simulink model "d_009_2"  (Simulink 8.3)
settings: Solver=ode45  StartTime=0.0  StopTime=10.0  RelTol=1e-3
libraries: fm_lib x9
settings Model: Creator=fmilano  LastModifiedBy=F  ExtModeAutoUpdateStatusClock=off
settings OptimizationCC: BooleanDataType=off  InitFltsAndDblsToZero=on
settings DebuggingCC: SaveWithParameterizedLinksMsg=none  SignalResolutionControl=TryResolveAllWithWarning  SolverPrmCheckMsg=none  MultiTaskDSMMsg=warning  MultiTaskCondExecSysMsg=none  StateNameClashWarn=none  StrictBusMsg=None
settings HardwareCC: TargetUnknown=on
settings RTWCC: IncludeERTFirstTime=on
settings GRTTargetCC: TargetFcnLib=ansi_tfl_tmw.mat  CodeReplacementLibrary=ANSI_C  CompOptLevelCompliant=off  CPPClassGenCompliant=off

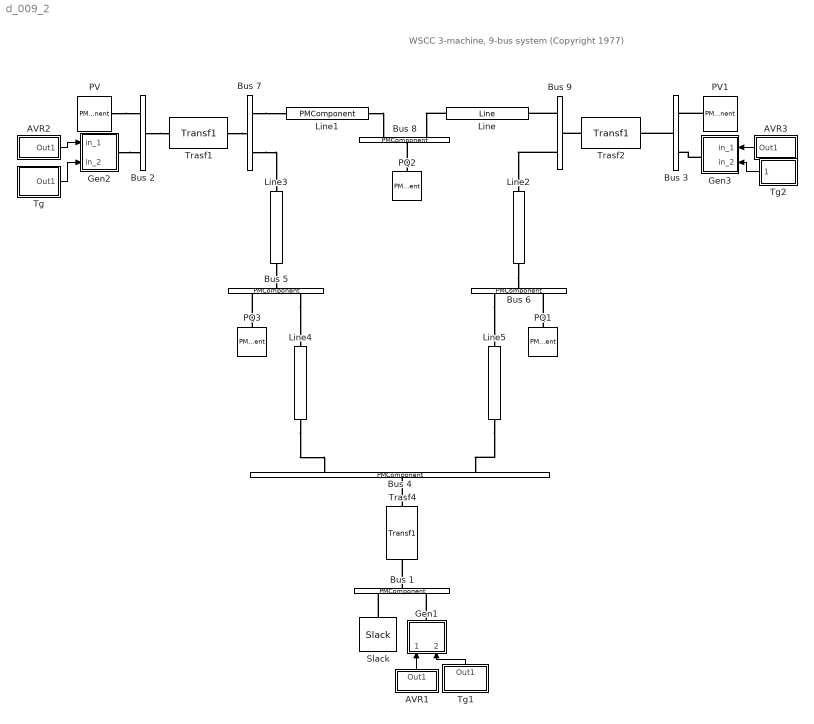
== system d_009_2 ==
  note: WSCC 3-machine, 9-bus system (Copyright 1977)
  AVR1 : Subsystem  Tag=PSATblock  Description=Controls  mask(Exc){p2q=2, p3q=5.00, p4q=-5.00, p5q=20, p6q=0.2, p7q=0.063, p8q=0.35, p9q=1, p10q=0.314, p11q=0.001, p12_13q=[0.0039  1.555], in=0}
      mask prompts: p2q "Automatic Voltage Regulator Type"; p3q "Maximum Regulator Voltage [p.u.]"; p4q "Minimum Regulator Voltage [p.u.]"; p5q "Amplifier Gain Ka [p.u./p.u.]"; p6q "Amplifier Time Constant Ta [s]"; p7q "Stabilizer Gain Kf [p.u./p.u.]"; p8q "Stabilizer Time Tf [s]"; p9q "Coefficient Kd [p.u./p.u.]"; p10q "Time Constant of the Field Circuit Td [s]"; p11q "Time Delay of the Measurement System Tr [s]"; p12_13q "Coefficient of the Ceiling Function (A B)"; in "Number of input signals"
      mask help: This block defines an Automatic Voltage Regulator.
      mask init:
      | fm_inout
      | [x,y] = fm_draw('R');
      mask Help:
      | This block defines an Automatic Voltage Regulator.
      | There are three kind of regulators:
      | 
      | Type 1:
      | 
      |      IEEE Model 1
      | 
      | Type 2:
      | 
      |      IEEE Model 2
      | 
      | Type 3:
      | 
      |      IEEE Model 3
      mask TypeOptions p2q: 1 | 2 | 3
      mask Callback p2q: fm_block
      mask TypeOptions in: 0 | 1 | 2 | 3
      mask Display:
      | plot([-1.8 4.1 4.1 -1.8 -1.8],[-1.5 -1.5 1.5 1.5 -1.5])
      | color('red')
      | plot([-1.3 -0.5],[-1 1],[-0.5 0.3],[1 -1],[-0.9 -0.1],[0.0 0.0])
      | plot(2.8+1.3*x,2*y,1.5+[-1.3 -0.5],[1 -1],1.5+[-0.5 0.3],[-1 1])
  AVR2 : Subsystem  Tag=PSATblock  Description=Controls  mask(Exc){p2q=2, p3q=5.00, p4q=-5.00, p5q=20, p6q=0.2, p7q=0.063, p8q=0.35, p9q=1, p10q=0.314, p11q=0.001, p12_13q=[0.0039  1.555], in=0}
      mask prompts: p2q "Automatic Voltage Regulator Type"; p3q "Maximum Regulator Voltage [p.u.]"; p4q "Minimum Regulator Voltage [p.u.]"; p5q "Amplifier Gain Ka [p.u./p.u.]"; p6q "Amplifier Time Constant Ta [s]"; p7q "Stabilizer Gain Kf [p.u./p.u.]"; p8q "Stabilizer Time Tf [s]"; p9q "Coefficient Kd [p.u./p.u.]"; p10q "Time Constant of the Field Circuit Td [s]"; p11q "Time Delay of the Measurement System Tr [s]"; p12_13q "Coefficient of the Ceiling Function (A B)"; in "Number of input signals"
      mask help: This block defines an Automatic Voltage Regulator.
      mask init:
      | fm_inout
      | [x,y] = fm_draw('R');
      mask Help:
      | This block defines an Automatic Voltage Regulator.
      | There are three kind of regulators:
      | 
      | Type 1:
      | 
      |      IEEE Model 1
      | 
      | Type 2:
      | 
      |      IEEE Model 2
      | 
      | Type 3:
      | 
      |      IEEE Model 3
      mask TypeOptions p2q: 1 | 2 | 3
      mask Callback p2q: fm_block
      mask TypeOptions in: 0 | 1 | 2 | 3
      mask Display:
      | plot([-1.8 4.1 4.1 -1.8 -1.8],[-1.5 -1.5 1.5 1.5 -1.5])
      | color('red')
      | plot([-1.3 -0.5],[-1 1],[-0.5 0.3],[1 -1],[-0.9 -0.1],[0.0 0.0])
      | plot(2.8+1.3*x,2*y,1.5+[-1.3 -0.5],[1 -1],1.5+[-0.5 0.3],[-1 1])
  AVR3 : Subsystem  Tag=PSATblock  Description=Controls  mask(Exc){p2q=2, p3q=5.00, p4q=-5.00, p5q=20, p6q=0.2, p7q=0.063, p8q=0.35, p9q=1, p10q=0.314, p11q=0.001, p12_13q=[0.0039  1.555], in=0}
      mask prompts: p2q "Automatic Voltage Regulator Type"; p3q "Maximum Regulator Voltage [p.u.]"; p4q "Minimum Regulator Voltage [p.u.]"; p5q "Amplifier Gain Ka [p.u./p.u.]"; p6q "Amplifier Time Constant Ta [s]"; p7q "Stabilizer Gain Kf [p.u./p.u.]"; p8q "Stabilizer Time Tf [s]"; p9q "Coefficient Kd [p.u./p.u.]"; p10q "Time Constant of the Field Circuit Td [s]"; p11q "Time Delay of the Measurement System Tr [s]"; p12_13q "Coefficient of the Ceiling Function (A B)"; in "Number of input signals"
      mask help: This block defines an Automatic Voltage Regulator.
      mask init:
      | fm_inout
      | [x,y] = fm_draw('R');
      mask Help:
      | This block defines an Automatic Voltage Regulator.
      | There are three kind of regulators:
      | 
      | Type 1:
      | 
      |      IEEE Model 1
      | 
      | Type 2:
      | 
      |      IEEE Model 2
      | 
      | Type 3:
      | 
      |      IEEE Model 3
      mask TypeOptions p2q: 1 | 2 | 3
      mask Callback p2q: fm_block
      mask TypeOptions in: 0 | 1 | 2 | 3
      mask Display:
      | plot([-1.8 4.1 4.1 -1.8 -1.8],[-1.5 -1.5 1.5 1.5 -1.5])
      | color('red')
      | plot([-1.3 -0.5],[-1 1],[-0.5 0.3],[1 -1],[-0.9 -0.1],[0.0 0.0])
      | plot(2.8+1.3*x,2*y,1.5+[-1.3 -0.5],[1 -1],1.5+[-0.5 0.3],[-1 1])
  Bus 1 : PMComponent  Tag=PSATblock  Description=Connection  PhysicalDomain=psatdomain  LeftPortType=p1  RightPortType=p1  LConnTagsString=__newl0|__newl1  RConnTagsString=__newr0  mask(Bus){in=2, out=1, p2q=16.5, p3_4q=[1.00   0.00], p5q=4, p6q=1}
      mask prompts: in "Number of inputs:"; out "Number of outputs:"; p2q "Voltage Rating [kV]"; p3_4q "Voltage initial guess [p.u.  rad]"; p5q "Area number"; p6q "Region number"
      mask help: Bus block.
      mask init:
      | fm_inout
      mask Callback p5q: fm_block
      mask Display: plot([0 1 1 0 0],[0 0 1 1 0])
  Bus 2 : PMComponent  Tag=PSATblock  Description=Connection  PhysicalDomain=psatdomain  LeftPortType=p1  RightPortType=p1  LConnTagsString=__newl0|__newl1  RConnTagsString=__newr0  mask(Bus){in=2, out=1, p2q=18, p3_4q=[1.00   0.00], p5q=5, p6q=1}
      mask prompts: in "Number of inputs:"; out "Number of outputs:"; p2q "Voltage Rating [kV]"; p3_4q "Voltage initial guess [p.u.  rad]"; p5q "Area number"; p6q "Region number"
      mask help: Bus block.
      mask init:
      | fm_inout
      mask Callback p5q: fm_block
      mask Display: plot([0 1 1 0 0],[0 0 1 1 0])
  Bus 3 : PMComponent  Tag=PSATblock  Description=Connection  PhysicalDomain=psatdomain  LeftPortType=p1  RightPortType=p1  LConnTagsString=__newl0|__newl1  RConnTagsString=__newr0  mask(Bus){in=2, out=1, p2q=13.8, p3_4q=[1.00   0.00], p5q=3, p6q=1}
      mask prompts: in "Number of inputs:"; out "Number of outputs:"; p2q "Voltage Rating [kV]"; p3_4q "Voltage initial guess [p.u.  rad]"; p5q "Area number"; p6q "Region number"
      mask help: Bus block.
      mask init:
      | fm_inout
      mask Callback p5q: fm_block
      mask Display: plot([0 1 1 0 0],[0 0 1 1 0])
  Bus 4 : PMComponent  Tag=PSATblock  Description=Connection  PhysicalDomain=psatdomain  LeftPortType=p1  RightPortType=p1  LConnTagsString=__newl0|__newl1  RConnTagsString=__newr0  mask(Bus){in=2, out=1, p2q=230, p3_4q=[1.00   0.00], p5q=2, p6q=1}
      mask prompts: in "Number of inputs:"; out "Number of outputs:"; p2q "Voltage Rating [kV]"; p3_4q "Voltage initial guess [p.u.  rad]"; p5q "Area number"; p6q "Region number"
      mask help: Bus block.
      mask init:
      | fm_inout
      mask Callback p5q: fm_block
      mask Display: plot([0 1 1 0 0],[0 0 1 1 0])
  Bus 5 : PMComponent  Tag=PSATblock  Description=Connection  PhysicalDomain=psatdomain  LeftPortType=p1  RightPortType=p1  LConnTagsString=__newl0  RConnTagsString=__newr0|__newr1  mask(Bus){in=1, out=2, p2q=230, p3_4q=[1.00   0.00], p5q=2, p6q=1}
      mask prompts: in "Number of inputs:"; out "Number of outputs:"; p2q "Voltage Rating [kV]"; p3_4q "Voltage initial guess [p.u.  rad]"; p5q "Area number"; p6q "Region number"
      mask help: Bus block.
      mask init:
      | fm_inout
      mask Callback p5q: fm_block
      mask Display: plot([0 1 1 0 0],[0 0 1 1 0])
  Bus 6 : PMComponent  Tag=PSATblock  Description=Connection  PhysicalDomain=psatdomain  LeftPortType=p1  RightPortType=p1  LConnTagsString=__newl0  RConnTagsString=__newr0|__newr1  mask(Bus){in=1, out=2, p2q=230, p3_4q=[1.00   0.00], p5q=2, p6q=1}
      mask prompts: in "Number of inputs:"; out "Number of outputs:"; p2q "Voltage Rating [kV]"; p3_4q "Voltage initial guess [p.u.  rad]"; p5q "Area number"; p6q "Region number"
      mask help: Bus block.
      mask init:
      | fm_inout
      mask Callback p5q: fm_block
      mask Display: plot([0 1 1 0 0],[0 0 1 1 0])
  Bus 7 : PMComponent  Tag=PSATblock  Description=Connection  PhysicalDomain=psatdomain  LeftPortType=p1  RightPortType=p1  LConnTagsString=__newl0  RConnTagsString=__newr0|__newr1  mask(Bus){in=1, out=2, p2q=230, p3_4q=[1.00   0.00], p5q=2, p6q=1}
      mask prompts: in "Number of inputs:"; out "Number of outputs:"; p2q "Voltage Rating [kV]"; p3_4q "Voltage initial guess [p.u.  rad]"; p5q "Area number"; p6q "Region number"
      mask help: Bus block.
      mask init:
      | fm_inout
      mask Callback p5q: fm_block
      mask Display: plot([0 1 1 0 0],[0 0 1 1 0])
  Bus 8 : PMComponent  Tag=PSATblock  Description=Connection  PhysicalDomain=psatdomain  LeftPortType=p1  RightPortType=p1  LConnTagsString=__newl0|__newl1  RConnTagsString=__newr0  mask(Bus){in=2, out=1, p2q=230, p3_4q=[1.00   0.00], p5q=2, p6q=1}
      mask prompts: in "Number of inputs:"; out "Number of outputs:"; p2q "Voltage Rating [kV]"; p3_4q "Voltage initial guess [p.u.  rad]"; p5q "Area number"; p6q "Region number"
      mask help: Bus block.
      mask init:
      | fm_inout
      mask Callback p5q: fm_block
      mask Display: plot([0 1 1 0 0],[0 0 1 1 0])
  Bus 9 : PMComponent  Tag=PSATblock  Description=Connection  PhysicalDomain=psatdomain  LeftPortType=p1  RightPortType=p1  LConnTagsString=__newl0  RConnTagsString=__newr0|__newr1  mask(Bus){in=1, out=2, p2q=230, p3_4q=[1.00   0.00], p5q=2, p6q=1}
      mask prompts: in "Number of inputs:"; out "Number of outputs:"; p2q "Voltage Rating [kV]"; p3_4q "Voltage initial guess [p.u.  rad]"; p5q "Area number"; p6q "Region number"
      mask help: Bus block.
      mask init:
      | fm_inout
      mask Callback p5q: fm_block
      mask Display: plot([0 1 1 0 0],[0 0 1 1 0])
  Gen1 : Subsystem  Tag=PSATblock  Description=Machines  mask(Syn){p2_3_4q=[100  16.5   60], p5q=4, p7_6q=[0.00  0.00], p8_9_10q=[0.1460  0.0608  0.0000], p11_12q=[8.96  0.00], p13_14_15q=[0.0969  0.0969  0.0000], p16_17q=[0.310  0.0000], p18_19q=[22  0.00], p20_21q=[0.00  0.00], p22_23q=[1.00  1.00], p24q=0.002, p25_26q=[0 0], in=2, p27q=1, p28q=on}
      mask prompts: p2_3_4q "Power, voltage and frequency ratings [MVA, kV, Hz]"; p5q "Machine Dynamic Order"; p7_6q "resistance ra and leakage reactance xl [p.u. p.u.]"; p8_9_10q "d-axis reactances Xd, X'd X"d [p.u.,p.u.,p.u.]"; p11_12q "d-axis open circuit time constants T'd0 and T"d0 [s, s]"; p13_14_15q "q-axis reactances Xq, X'q, X"q [p.u.  p.u.  p.u.]"; p16_17q "q-axis open circuit time constants T'q0 and T"q0 [s s]"; p18_19q "Inertia (M = 2H) and Damping [s, p.u.]"; p20_21q "Speed and active power additional signals Kw and Kp [p.u., p.u.]"; p22_23q "Percentage of active and reactive powers at bus [p.u. p.u.]"; p24q "d-axis additional circuit leakage time constant Taa [s]"; p25_26q "Saturation coefficients S(1.0) and S(1.2)"; in "Number of input signals"; p27q "COI number"; p28q "Connected"
      mask help: This block defines a fourth order synchronous machine.
      mask init:
      | fm_inout
      | [x,y] = fm_draw('circle');
      | [xg,yg] = fm_draw('G');
      | [xs,ys] = fm_draw('sinus');
      mask TypeOptions p5q: 8 | 6 | 5.3 | 5.2 | 5.1 | 4 | 3 | 2
      mask Callback p5q: fm_block
      mask TypeOptions in: 0 | 1 | 2
      mask Callback p28q: fm_block
      mask Display:
      | plot(x+1.4,y,0.12*xs+1,0.15*ys-0.6)
      | color('blue')
      | plot(1.4+0.45*xg,0.3+0.45*yg)
  Gen2 : Subsystem  Tag=PSATblock  Description=Machines  mask(Syn){p2_3_4q=[100  18   60], p5q=4, p7_6q=[0.00  0.00], p8_9_10q=[0.8958  0.1198  0.0000], p11_12q=[6.00  0.00], p13_14_15q=[0.8645  0.1969  0.0000], p16_17q=[0.5350  0.0000], p18_19q=[22  0.00], p20_21q=[0.00  0.00], p22_23q=[1.00  1.00], p24q=0.002, p25_26q=[0 0], in=2, p27q=1, p28q=on}
      mask prompts: p2_3_4q "Power, voltage and frequency ratings [MVA, kV, Hz]"; p5q "Machine Dynamic Order"; p7_6q "resistance ra and leakage reactance xl [p.u. p.u.]"; p8_9_10q "d-axis reactances Xd, X'd X"d [p.u.,p.u.,p.u.]"; p11_12q "d-axis open circuit time constants T'd0 and T"d0 [s, s]"; p13_14_15q "q-axis reactances Xq, X'q, X"q [p.u.  p.u.  p.u.]"; p16_17q "q-axis open circuit time constants T'q0 and T"q0 [s s]"; p18_19q "Inertia (M = 2H) and Damping [s, p.u.]"; p20_21q "Speed and active power additional signals Kw and Kp [p.u., p.u.]"; p22_23q "Percentage of active and reactive powers at bus [p.u. p.u.]"; p24q "d-axis additional circuit leakage time constant Taa [s]"; p25_26q "Saturation coefficients S(1.0) and S(1.2)"; in "Number of input signals"; p27q "COI number"; p28q "Connected"
      mask help: This block defines a fourth order synchronous machine.
      mask init:
      | fm_inout
      | [x,y] = fm_draw('circle');
      | [xg,yg] = fm_draw('G');
      | [xs,ys] = fm_draw('sinus');
      mask TypeOptions p5q: 8 | 6 | 5.3 | 5.2 | 5.1 | 4 | 3 | 2
      mask Callback p5q: fm_block
      mask TypeOptions in: 0 | 1 | 2
      mask Callback p28q: fm_block
      mask Display:
      | plot(x+1.4,y,0.12*xs+1,0.15*ys-0.6)
      | color('blue')
      | plot(1.4+0.45*xg,0.3+0.45*yg)
  Gen3 : Subsystem  Tag=PSATblock  Description=Machines  mask(Syn){p2_3_4q=[100  13.8   60], p5q=4, p7_6q=[0.00  0.00], p8_9_10q=[1.3125  0.1813  0.0000], p11_12q=[5.89  0.00], p13_14_15q=[1.2578  0.2500  0.0000], p16_17q=[0.600  0.0000], p18_19q=[4.4  0.00], p20_21q=[0.00  0.00], p22_23q=[1.00  1.00], p24q=0.002, p25_26q=[0 0], in=2, p27q=1, p28q=on}
      mask prompts: p2_3_4q "Power, voltage and frequency ratings [MVA, kV, Hz]"; p5q "Machine Dynamic Order"; p7_6q "resistance ra and leakage reactance xl [p.u. p.u.]"; p8_9_10q "d-axis reactances Xd, X'd X"d [p.u.,p.u.,p.u.]"; p11_12q "d-axis open circuit time constants T'd0 and T"d0 [s, s]"; p13_14_15q "q-axis reactances Xq, X'q, X"q [p.u.  p.u.  p.u.]"; p16_17q "q-axis open circuit time constants T'q0 and T"q0 [s s]"; p18_19q "Inertia (M = 2H) and Damping [s, p.u.]"; p20_21q "Speed and active power additional signals Kw and Kp [p.u., p.u.]"; p22_23q "Percentage of active and reactive powers at bus [p.u. p.u.]"; p24q "d-axis additional circuit leakage time constant Taa [s]"; p25_26q "Saturation coefficients S(1.0) and S(1.2)"; in "Number of input signals"; p27q "COI number"; p28q "Connected"
      mask help: This block defines a fourth order synchronous machine.
      mask init:
      | fm_inout
      | [x,y] = fm_draw('circle');
      | [xg,yg] = fm_draw('G');
      | [xs,ys] = fm_draw('sinus');
      mask TypeOptions p5q: 8 | 6 | 5.3 | 5.2 | 5.1 | 4 | 3 | 2
      mask Callback p5q: fm_block
      mask TypeOptions in: 0 | 1 | 2
      mask Callback p28q: fm_block
      mask Display:
      | plot(x+1.4,y,0.12*xs+1,0.15*ys-0.6)
      | color('blue')
      | plot(1.4+0.45*xg,0.3+0.45*yg)
  Line : fm_lib/Power Flow/Line  Tag=PSATblock  Description=Power Flow  LConnTagsString=__newl0  RConnTagsString=__newr0  p3_4_5q="[100  230  60]"  p6q=0  p8q=0.0119  p9q=0.1008  p10q=0.1045*2  p13_14_15q="[0.0  0.0  0.0]"  p16q=on
  Line1 : PMComponent  Tag=PSATblock  Description=Power Flow  PhysicalDomain=psatdomain  LeftPortType=p1  RightPortType=p1  LConnTagsString=__newl0  RConnTagsString=__newr0  mask(Line){p3_4_5q=[100  230  60], p6q=0, p8q=0.0085, p9q=0.072, p10q=0.0745*2, p13_14_15q=[0.0  0.0  0.0], p16q=on}
      mask prompts: p3_4_5q "Power, Voltage and Frequency Ratings [MVA, kV, Hz]"; p6q "Length of line [km] (0 for p.u. parameters)"; p8q "Resistance [p.u. (Ohms/km)]"; p9q "Reactance [p.u. (H/km)]"; p10q "Susceptance [p.u. (F/km)]"; p13_14_15q "Imax, Pmax and Smax [p.u., p.u., p.u.]"; p16q "Connected"
      mask help: This block defines a pi model for a tree phase line.
      mask init:
      | [xp,yp] = fm_draw('pi');
      mask Callback p16q: fm_block
      mask Display:
      | plot([-1  1  1 -1 -1],[-0.2 -0.2 0.2 0.2 -0.2])
      | color('blue')
      | plot(0.35*xp,0.2*yp)
  Line2 : fm_lib/Power Flow/Line  Tag=PSATblock  Description=Power Flow  LConnTagsString=__newl0  RConnTagsString=__newr0  p3_4_5q="[100  230  60]"  p6q=0  p8q=0.039  p9q=0.170  p10q=0.179*2  p13_14_15q="[0.0  0.0  0.0]"  p16q=on
  Line3 : fm_lib/Power Flow/Line  Tag=PSATblock  Description=Power Flow  LConnTagsString=__newl0  RConnTagsString=__newr0  p3_4_5q="[100  230  60]"  p6q=0  p8q=0.032  p9q=0.161  p10q=0.153*2  p13_14_15q="[0.0  0.0  0.0]"  p16q=on
  Line4 : fm_lib/Power Flow/Line  Tag=PSATblock  Description=Power Flow  LConnTagsString=__newl0  RConnTagsString=__newr0  p3_4_5q="[100  230  60]"  p6q=0  p8q=0.01  p9q=0.085  p10q=0.088*2  p13_14_15q="[0.0  0.0  0.0]"  p16q=on
  Line5 : fm_lib/Power Flow/Line  Tag=PSATblock  Description=Power Flow  LConnTagsString=__newl0  RConnTagsString=__newr0  p3_4_5q="[100  230  60]"  p6q=0  p8q=0.017  p9q=0.092  p10q=0.079*2  p13_14_15q="[0.0  0.0  0.0]"  p16q=on
  PQ1 : PMComponent  Tag=PSATblock  Description=Power Flow  PhysicalDomain=psatdomain  LeftPortType=p1  RightPortType=p1  LConnTagsString=__newl0  mask(PQ){p2_3q=[100  230], p4_5q=[0.9  0.3], p6_7q=[1.2  0.8], p8q=off, p9q=on}
      mask prompts: p2_3q "Power and Voltage Ratings [MVA, kV]"; p4_5q "Active and Reactive Powers [p.u.  p.u.]"; p6_7q "Maximum and Minimum Allowable Voltage [p.u.   p.u.]"; p8q "Allow conversion to impendance for min & max voltage"; p9q "Connected"
      mask help:
      | This block defines a constant power load:
      |
      | P = Pcost.
      | Q = Qcost.
      mask Callback p8q: fm_block
      mask Callback p9q: fm_block
      mask Display: plot([1 -0.5 -0.5 1],[0 0.866 -0.866 0])
  PQ2 : PMComponent  Tag=PSATblock  Description=Power Flow  PhysicalDomain=psatdomain  LeftPortType=p1  RightPortType=p1  LConnTagsString=__newl0  mask(PQ){p2_3q=[100  230], p4_5q=[1  0.35], p6_7q=[1.2  0.8], p8q=off, p9q=on}
      mask prompts: p2_3q "Power and Voltage Ratings [MVA, kV]"; p4_5q "Active and Reactive Powers [p.u.  p.u.]"; p6_7q "Maximum and Minimum Allowable Voltage [p.u.   p.u.]"; p8q "Allow conversion to impendance for min & max voltage"; p9q "Connected"
      mask help:
      | This block defines a constant power load:
      |
      | P = Pcost.
      | Q = Qcost.
      mask Callback p8q: fm_block
      mask Callback p9q: fm_block
      mask Display: plot([1 -0.5 -0.5 1],[0 0.866 -0.866 0])
  PQ3 : PMComponent  Tag=PSATblock  Description=Power Flow  PhysicalDomain=psatdomain  LeftPortType=p1  RightPortType=p1  LConnTagsString=__newl0  mask(PQ){p2_3q=[100  230], p4_5q=[1.25  0.5], p6_7q=[1.2  0.8], p8q=off, p9q=on}
      mask prompts: p2_3q "Power and Voltage Ratings [MVA, kV]"; p4_5q "Active and Reactive Powers [p.u.  p.u.]"; p6_7q "Maximum and Minimum Allowable Voltage [p.u.   p.u.]"; p8q "Allow conversion to impendance for min & max voltage"; p9q "Connected"
      mask help:
      | This block defines a constant power load:
      |
      | P = Pcost.
      | Q = Qcost.
      mask Callback p8q: fm_block
      mask Callback p9q: fm_block
      mask Display: plot([1 -0.5 -0.5 1],[0 0.866 -0.866 0])
  PV : PMComponent  Tag=PSATblock  Description=Power Flow  PhysicalDomain=psatdomain  LeftPortType=p1  RightPortType=p1  RConnTagsString=__newr0  mask(PV){p2_3q=[100  18], p4q=1.316, p5q=1.025, p6_7q=[99 -99], p8_9q=[1.1  0.9], p10q=1, p11q=on}
      mask prompts: p2_3q "Power and Voltage Ratings [MVA, kV]"; p4q "Active Power [p.u.]"; p5q "Voltage Magnitude [p.u.]"; p6_7q "Qmax and Qmin [p.u.  p.u.]"; p8_9q "Vmax and Vmin [p.u.  p.u.]"; p10q "Loss Participation Factor"; p11q "Connected"
      mask help:
      | This block defines a PV bus for load flow studies:
      |
      | P = Pcost.
      | V = Vdes.
      mask init:
      | [x,y] = fm_draw('circle');
      | [xp,yp] = fm_draw('P');
      mask Callback p11q: fm_block
      mask Display:
      | plot(x,y)
      | color('blue')
      | plot(0.3*xp-0.35,0.6*yp,[0.1 0.3 0.5],[0.3 -0.3 0.3])
  PV1 : PMComponent  Tag=PSATblock  Description=Power Flow  PhysicalDomain=psatdomain  LeftPortType=p1  RightPortType=p1  RConnTagsString=__newr0  mask(PV){p2_3q=[100  13.8], p4q=1.162, p5q=1.025, p6_7q=[99  -99], p8_9q=[1.1  0.9], p10q=1, p11q=on}
      mask prompts: p2_3q "Power and Voltage Ratings [MVA, kV]"; p4q "Active Power [p.u.]"; p5q "Voltage Magnitude [p.u.]"; p6_7q "Qmax and Qmin [p.u.  p.u.]"; p8_9q "Vmax and Vmin [p.u.  p.u.]"; p10q "Loss Participation Factor"; p11q "Connected"
      mask help:
      | This block defines a PV bus for load flow studies:
      |
      | P = Pcost.
      | V = Vdes.
      mask init:
      | [x,y] = fm_draw('circle');
      | [xp,yp] = fm_draw('P');
      mask Callback p11q: fm_block
      mask Display:
      | plot(x,y)
      | color('blue')
      | plot(0.3*xp-0.35,0.6*yp,[0.1 0.3 0.5],[0.3 -0.3 0.3])
  Slack : fm_lib/Power Flow/Slack  Tag=PSATblock  Description=Power Flow  RConnTagsString=__newr0  p2_3q="[100  16.5]"  p4q=1.04  p5q=0.00  p6_7q=[99 -99]  p8_9q="[1.1  0.9]"  p10q=0.80  p11q=1  p12q=on  p13q=on
  Tg : Subsystem  Tag=PSATblock  Description=Controls  mask(Tg){p2q=2, p3q=1.00, p4q=0.2, p5q=10, p6q=0.0, p7q=0.10, p8q=-0.10, p9q=0.04, p10q=5.0, p11q=0.04, p12q=0.3, p13q=1.0, p14q=0.5, p15q=1.0, p16q=1.5, p17q=1.0, p18q=1.163, p19q=0.105, p20q=on}
      mask prompts: p2q "Turbine governor type"; p3q "Reference speed [p.u.]"; p4q "Droop R [p.u.]"; p5q "Maximum torque [p.u.]"; p6q "Minimum torque [p.u.]"; p7q "Pole Time Constant T2 [s]"; p8q "Zero Time Constant T1 [s]"; p9q "Pilot valve time constant Tp [s]"; p10q "Dashpot time constant Tr [s]"; p11q "Permanent speed droop sigma [p.u./p.u.]"; p12q "Transient speed droop delta [p.u./p.u.]"; p13q "Water starting time Tw [s]"; p14q "Derivative of flow rate with respect to tubine head a11"; p15q "Derivative of flow rate with respect to gate position a13"; p16q "Derivative of torque with respect to tubine head a21"; p17q "Derivative of torque with respect to gate position a23"; p18q "Proportional droop Kp [p.u./p.u.]"; p19q "Integral droop Ki [p.u./p.u.]"; p20q "Connected"
      mask help: This block defines a Turbine Governor.
      mask init:
      | [x,y] = fm_draw('G');
      mask TypeOptions p2q: 1 | 2 | 3 | 4 | 5 | 6
      mask Callback p2q: fm_block
      mask Callback p20q: fm_block
      mask Display:
      | plot([-1.8 2.8 2.8 -1.8 -1.8],[-1.5 -1.5 1.5 1.5 -1.5])
      | color('red')
      | plot([-0.5 -0.5],[-1 1],[-1.3 0.3],[1 1])
      | plot(1.4+x,y)
  Tg1 : Subsystem  Tag=PSATblock  Description=Controls  mask(Tg){p2q=2, p3q=1.00, p4q=0.2, p5q=10, p6q=0.0, p7q=0.10, p8q=-0.10, p9q=0.04, p10q=5.0, p11q=0.04, p12q=0.3, p13q=1.0, p14q=0.5, p15q=1.0, p16q=1.5, p17q=1.0, p18q=1.163, p19q=0.105, p20q=on}
      mask prompts: p2q "Turbine governor type"; p3q "Reference speed [p.u.]"; p4q "Droop R [p.u.]"; p5q "Maximum torque [p.u.]"; p6q "Minimum torque [p.u.]"; p7q "Pole Time Constant T2 [s]"; p8q "Zero Time Constant T1 [s]"; p9q "Pilot valve time constant Tp [s]"; p10q "Dashpot time constant Tr [s]"; p11q "Permanent speed droop sigma [p.u./p.u.]"; p12q "Transient speed droop delta [p.u./p.u.]"; p13q "Water starting time Tw [s]"; p14q "Derivative of flow rate with respect to tubine head a11"; p15q "Derivative of flow rate with respect to gate position a13"; p16q "Derivative of torque with respect to tubine head a21"; p17q "Derivative of torque with respect to gate position a23"; p18q "Proportional droop Kp [p.u./p.u.]"; p19q "Integral droop Ki [p.u./p.u.]"; p20q "Connected"
      mask help: This block defines a Turbine Governor.
      mask init:
      | [x,y] = fm_draw('G');
      mask TypeOptions p2q: 1 | 2 | 3 | 4 | 5 | 6
      mask Callback p2q: fm_block
      mask Callback p20q: fm_block
      mask Display:
      | plot([-1.8 2.8 2.8 -1.8 -1.8],[-1.5 -1.5 1.5 1.5 -1.5])
      | color('red')
      | plot([-0.5 -0.5],[-1 1],[-1.3 0.3],[1 1])
      | plot(1.4+x,y)
  Tg2 : Subsystem  Tag=PSATblock  Description=Controls  mask(Tg){p2q=2, p3q=1.00, p4q=0.2, p5q=10, p6q=0.0, p7q=0.10, p8q=-0.10, p9q=0.04, p10q=5.0, p11q=0.04, p12q=0.3, p13q=1.0, p14q=0.5, p15q=1.0, p16q=1.5, p17q=1.0, p18q=1.163, p19q=0.105, p20q=on}
      mask prompts: p2q "Turbine governor type"; p3q "Reference speed [p.u.]"; p4q "Droop R [p.u.]"; p5q "Maximum torque [p.u.]"; p6q "Minimum torque [p.u.]"; p7q "Pole Time Constant T2 [s]"; p8q "Zero Time Constant T1 [s]"; p9q "Pilot valve time constant Tp [s]"; p10q "Dashpot time constant Tr [s]"; p11q "Permanent speed droop sigma [p.u./p.u.]"; p12q "Transient speed droop delta [p.u./p.u.]"; p13q "Water starting time Tw [s]"; p14q "Derivative of flow rate with respect to tubine head a11"; p15q "Derivative of flow rate with respect to gate position a13"; p16q "Derivative of torque with respect to tubine head a21"; p17q "Derivative of torque with respect to gate position a23"; p18q "Proportional droop Kp [p.u./p.u.]"; p19q "Integral droop Ki [p.u./p.u.]"; p20q "Connected"
      mask help: This block defines a Turbine Governor.
      mask init:
      | [x,y] = fm_draw('G');
      mask TypeOptions p2q: 1 | 2 | 3 | 4 | 5 | 6
      mask Callback p2q: fm_block
      mask Callback p20q: fm_block
      mask Display:
      | plot([-1.8 2.8 2.8 -1.8 -1.8],[-1.5 -1.5 1.5 1.5 -1.5])
      | color('red')
      | plot([-0.5 -0.5],[-1 1],[-1.3 0.3],[1 1])
      | plot(1.4+x,y)
  Trasf1 : fm_lib/Power Flow/Transf1  Tag=PSATblock  Description=Power Flow  LConnTagsString=__newl0  RConnTagsString=__newr0  p3_4_5q="[100  18  60]"  p7q=18/230  p8q=0.0  p9q=0.0625  p13_14_15q="[0.0  0.0  0.0]"  p16q=on
  Trasf2 : fm_lib/Power Flow/Transf1  Tag=PSATblock  Description=Power Flow  LConnTagsString=__newl0  RConnTagsString=__newr0  p3_4_5q="[100  13.8  60]"  p7q=13.8/230  p8q=0.0  p9q=0.0586  p13_14_15q="[0.0  0.0  0.0]"  p16q=on
  Trasf4 : fm_lib/Power Flow/Transf1  Tag=PSATblock  Description=Power Flow  LConnTagsString=__newl0  RConnTagsString=__newr0  p3_4_5q="[100  16.5  60]"  p7q=16.5/230  p8q=0.0  p9q=0.0576  p13_14_15q="[0.0  0.0  0.0]"  p16q=on
  wires:
  AVR2/1(Out1) -> Gen2/1(in_1)
  AVR3/1(Out1) -> Gen3/1(in_1)
  AVR1/1(Out1) -> Gen1/1(in_1)
  Tg/1(Out1) -> Gen2/2(in_2)
  Tg1/1(Out1) -> Gen1/2(in_2)
  Tg2/1(Out1) -> Gen3/2(in_2)
  connections:
  Gen3/RConn1 -- Bus 3/LConn2
  Gen2/RConn1 -- Bus 2/LConn2
  Line5/RConn1 -- Bus 4/LConn2
  Line4/RConn1 -- Bus 4/LConn1
  Bus 5/RConn2 -- Line4/LConn1
  Bus 6/RConn1 -- Line5/LConn1
  Line3/RConn1 -- Bus 5/LConn1
  Line2/RConn1 -- Bus 6/LConn1
  Bus 9/RConn2 -- Line2/LConn1
  Line/RConn1 -- Bus 8/LConn2
  Bus 7/RConn1 -- Line1/LConn1
  Bus 9/RConn1 -- Line/LConn1
  Trasf2/RConn1 -- Bus 9/LConn1
  Trasf1/RConn1 -- Bus 7/LConn1
  Bus 3/RConn1 -- Trasf2/LConn1
  Bus 2/RConn1 -- Trasf1/LConn1
  PV1/RConn1 -- Bus 3/LConn1
  PV/RConn1 -- Bus 2/LConn1
  PQ1/LConn1 -- Bus 6/RConn2
  PQ2/LConn1 -- Bus 8/RConn1
  PQ3/LConn1 -- Bus 5/RConn1
  Line1/RConn1 -- Bus 8/LConn1
  Trasf4/RConn1 -- Bus 4/RConn1
  Bus 1/RConn1 -- Trasf4/LConn1
  Slack/RConn1 -- Bus 1/LConn1
  Gen1/RConn1 -- Bus 1/LConn2
  Bus 7/RConn2 -- Line3/LConn1

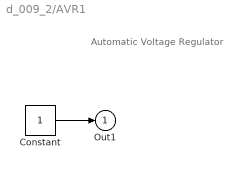
== system d_009_2/AVR1 ==
  note: Automatic Voltage Regulator
  Constant : Constant
  Out1 : Outport
  wires:
  Constant/1 -> Out1/1

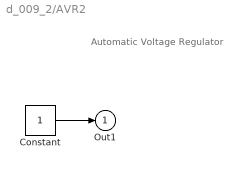
== system d_009_2/AVR2 ==
  note: Automatic Voltage Regulator
  Constant : Constant
  Out1 : Outport
  wires:
  Constant/1 -> Out1/1

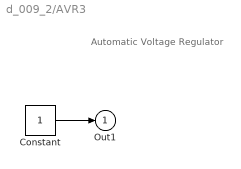
== system d_009_2/AVR3 ==
  note: Automatic Voltage Regulator
  Constant : Constant
  Out1 : Outport
  wires:
  Constant/1 -> Out1/1

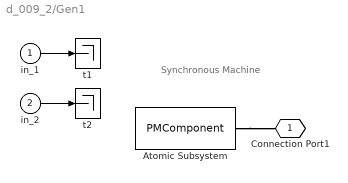
== system d_009_2/Gen1 ==
  note: Synchronous Machine
  in_1 : Inport
  in_2 : Inport  Port=2
  Atomic Subsystem : PMComponent  PhysicalDomain=psatdomain  LeftPortType=p1  RightPortType=p1  RConnTagsString=__newr0
  t1 : Terminator
  t2 : Terminator
  Connection Port1 : PMIOPort  Tag=PMCPort  Port=1  Side=Right
  wires:
  in_1/1 -> t1/1
  in_2/1 -> t2/1
  connections:
  Atomic Subsystem/RConn1 -- Connection Port1/RConn1

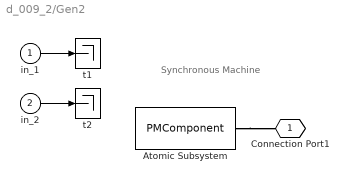
== system d_009_2/Gen2 ==
  note: Synchronous Machine
  in_1 : Inport
  in_2 : Inport  Port=2
  Atomic Subsystem : PMComponent  PhysicalDomain=psatdomain  LeftPortType=p1  RightPortType=p1  RConnTagsString=__newr0
  t1 : Terminator
  t2 : Terminator
  Connection Port1 : PMIOPort  Tag=PMCPort  Port=1  Side=Right
  wires:
  in_1/1 -> t1/1
  in_2/1 -> t2/1
  connections:
  Atomic Subsystem/RConn1 -- Connection Port1/RConn1

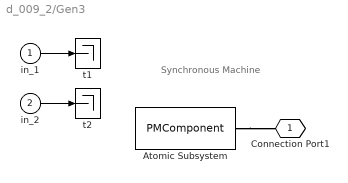
== system d_009_2/Gen3 ==
  note: Synchronous Machine
  in_1 : Inport
  in_2 : Inport  Port=2
  Atomic Subsystem : PMComponent  PhysicalDomain=psatdomain  LeftPortType=p1  RightPortType=p1  RConnTagsString=__newr0
  t1 : Terminator
  t2 : Terminator
  Connection Port1 : PMIOPort  Tag=PMCPort  Port=1  Side=Right
  wires:
  in_1/1 -> t1/1
  in_2/1 -> t2/1
  connections:
  Atomic Subsystem/RConn1 -- Connection Port1/RConn1

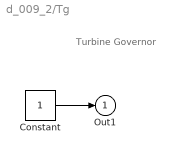
== system d_009_2/Tg ==
  note: Turbine Governor
  Constant : Constant
  Out1 : Outport
  wires:
  Constant/1 -> Out1/1

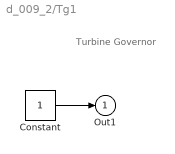
== system d_009_2/Tg1 ==
  note: Turbine Governor
  Constant : Constant
  Out1 : Outport
  wires:
  Constant/1 -> Out1/1

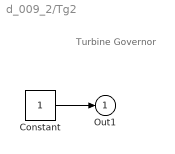
== system d_009_2/Tg2 ==
  note: Turbine Governor
  Constant : Constant
  Out1 : Outport
  wires:
  Constant/1 -> Out1/1
